simulink subsystem "Reference_curcle_trajectory"  (R2023b)
settings: Solver=VariableStepAuto  StartTime=0.0  StopTime=10.0  RelTol=1e-3
undefined symbols (not defined in the file): circile_ref_amplitude, circile_ref_frequency, MPC_PredictionHorizon, TimeStep_MPC
settings Model: Creator=tshintai  LastModifiedBy=tshintai
settings OptimizationCC: ReuseModelBlockBuffer=off
settings ModelReferenceCC: EnableRefExpFcnMdlSchedulingChecks=on

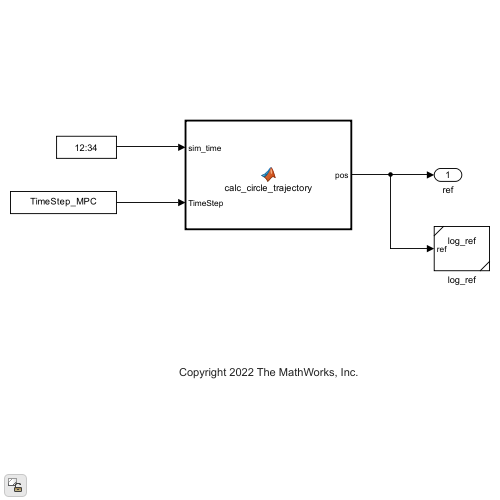
[thumbnail: Simulink's stored preview of the top-level diagram]
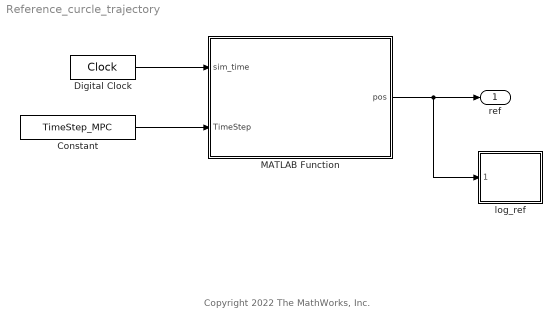
== system Reference_curcle_trajectory ==
  note: Copyright 2022 The MathWorks, Inc.
  Constant : Constant  Value=TimeStep_MPC
  Digital Clock : DigitalClock  SampleTime=TimeStep_MPC
  MATLAB Function : MATLAB Function  TreatAsAtomicUnit=on
  log_ref : Subsystem  ReferencedSubsystem=log_ref
  ref : Outport
  wires:
  MATLAB Function/1(pos) -> log_ref/1, ref/1
  Digital Clock/1 -> MATLAB Function/1(sim_time)
  Constant/1 -> MATLAB Function/2(TimeStep)

== matlab function Reference_curcle_trajectory/MATLAB Function ==
  data: sim_time input; pos output; circile_ref_frequency parameter; circile_ref_amplitude parameter; TimeStep input; MPC_PredictionHorizon parameter
function pos = calc_circle_trajectory(sim_time, circile_ref_frequency, ...
    circile_ref_amplitude, TimeStep, MPC_PredictionHorizon)
%%
pos = zeros(2, MPC_PredictionHorizon);


%%
for i = 0:(MPC_PredictionHorizon - 1)
    pos(1, i+1) = circile_ref_amplitude * sin(circile_ref_frequency * ...
        (sim_time + i*TimeStep) * 2*pi);
    pos(2, i+1) = circile_ref_amplitude * cos(circile_ref_frequency * ...
        (sim_time + i*TimeStep) * 2*pi);
end

end
